simulink subsystem "InversePendulum"  (R2023a)
settings: Solver=VariableStepAuto  StartTime=0.0  StopTime=10.0  RelTol=1e-3
values from neighbouring files (symbols this model uses):
  A = [0      1              0           0;      0      0          (m^2*g*l^2)/p   0;      0      0              0           1;      0      0          -m*g*l*(M+m)/p  0]    [InversePendulum_constant.m]
  B = [     0 ... (first row only)    [InversePendulum_constant.m]
  g = 9.8    [InversePendulum_constant.m]
  I = (m * l^2)/3    (= 0.00833333333333)    [InversePendulum_constant.m]
  Init_St = [ 0 0 deg2rad(5) 0]    [InversePendulum_constant.m]
  l = 0.5    [InversePendulum_constant.m]
  m = 0.1    [InversePendulum_constant.m]
  M = 0.2    [InversePendulum_constant.m]
  p = I*(M+m)+M*m*l^2    (= 0.0075)    [InversePendulum_constant.m]
settings Model: Creator=Лиза  LastModifiedBy=romav

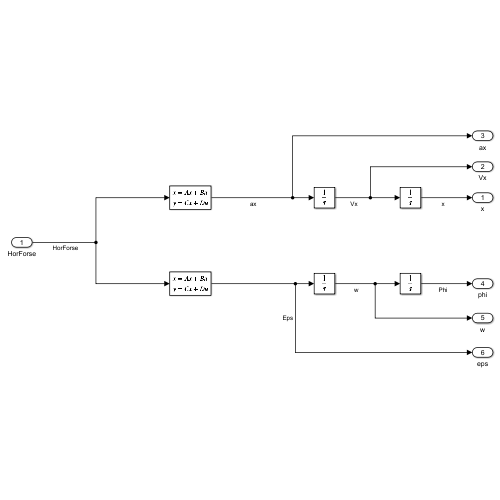
[thumbnail: Simulink's stored preview of the top-level diagram]
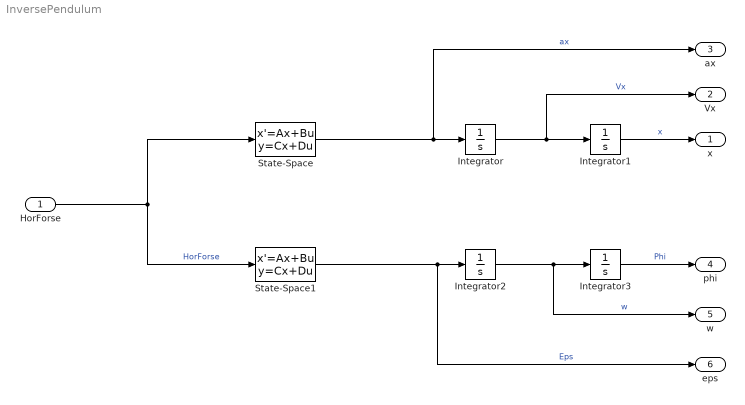
== system InversePendulum ==
  HorForse : Inport
  Integrator{,1..3} (4 alike) : Integrator
  State-Space : StateSpace  A=A  B=B  C="[ 0      0          (m^2*g*l^2)/p   0]"  D=[(I+m*l^2)/p]  InitialCondition=Init_St
  State-Space1 : StateSpace  A=A  B=B  C=[ 0 0 -m*g*l*(M+m)/p 0]  D=-m*l/p  InitialCondition=Init_St
  x : Outport
  Vx : Outport  Port=2
  ax : Outport  Port=3
  phi : Outport  Port=4
  w : Outport  Port=5
  eps : Outport  Port=6
  wires:
  HorForse/1 -> State-Space1/1, State-Space/1  "HorForse"
  State-Space/1 -> ax/1, Integrator/1  "ax"
  Integrator/1 -> Vx/1, Integrator1/1  "Vx"
  State-Space1/1 -> eps/1, Integrator2/1  "Eps"
  Integrator2/1 -> w/1, Integrator3/1  "w"
  Integrator1/1 -> x/1  "x"
  Integrator3/1 -> phi/1  "Phi"
